simulink model "VSMr_2023b"  (R2023b)
settings: Solver=ode14x  StartTime=0  StopTime=Sim.tend  FixedStep=0.000125  RelTol=4e-4
model workspace (MAT data in the model file):
  nr_vsm = Simulink.Parameter
  nr_vsm.Value = 2
  nr_vsm.DataType = 'int8'
  nr_vsm.Complexity = 'real'
  nr_vsm.Dimensions = [1 1]
values from neighbouring files (symbols this model uses):
  ControlSampleTime = 1/8000    (= 0.000125)    [sim3run_390.m]
  ddfmax = 60    [prm3var_390.m]
  T_seccontrol = 20    [prm3var_390.m]
  Ts = TS    [sim3run_390.m]
  TVRint = 0.85    [prm3var_390.m]
  vsm_Tdaco = 0.01    [prm3var_390.m]
undefined symbols (not defined in the file or in its folder): DiscIntNeverNeededParam, General, parameterset, prm_vsm, pu_vsm, UFLS, VSM
libraries: simulink x55, FriedrichLibrary x10, simulink_extras x2, spsSampleandHoldLib x2
(part 1 of 3)
settings Model: ParameterArgumentNames=nr_vsm  Creator=e2n052  LastModifiedBy=uk062294
settings SolverCC: AlgebraicLoopSolver=TrustRegion
settings DataIOCC: SaveOutput=off  SaveTime=off  ReturnWorkspaceOutputs=off
settings DebuggingCC: UnconnectedInputMsg=warning  UnconnectedOutputMsg=warning  UnconnectedLineMsg=warning  ArithmeticOperatorsInVariantConditions=warning
settings ModelReferenceCC: EnableRefExpFcnMdlSchedulingChecks=on
settings SFSimCC: SimUseLocalCustomCode=off  CustomCodeUndefinedFunction=UseInterfaceOnly
settings RTWCC: RTWUseLocalCustomCode=off  DLArmComputeVersion=19.05
settings GRTTargetCC: CombineOutputUpdateFcns=off  MatFileLogging=off

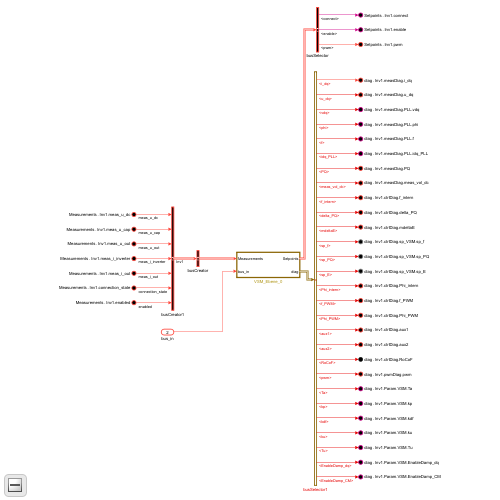
[thumbnail: Simulink's stored preview of the top-level diagram]
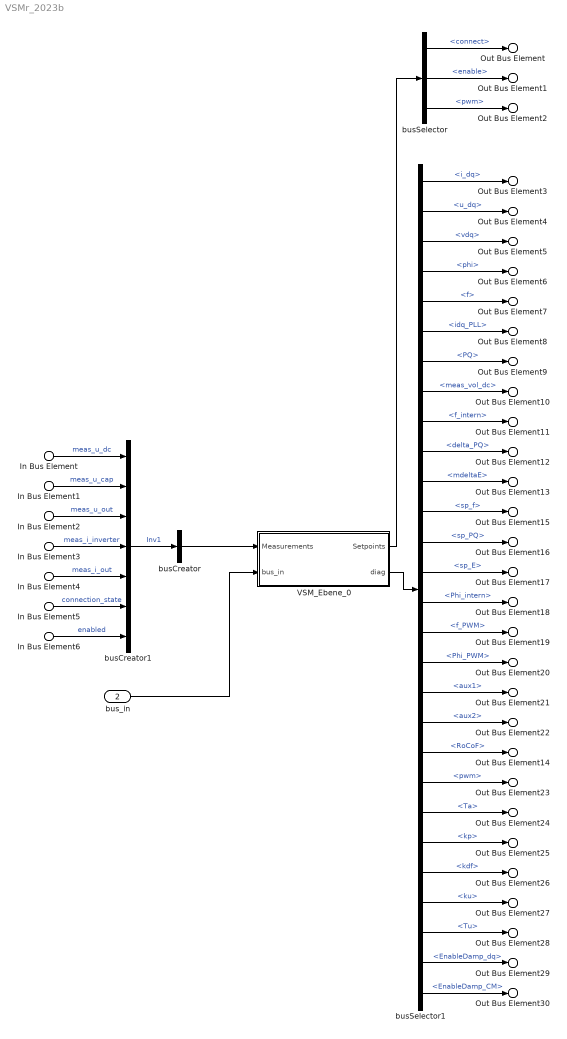
== system VSMr_2023b ==
  In Bus Element : Inport  PortName=Measurements  Element=Inv1.meas_u_dc
  In Bus Element1 : Inport  PortName=Measurements  Element=Inv1.meas_u_cap
  In Bus Element2 : Inport  PortName=Measurements  Element=Inv1.meas_u_out
  In Bus Element3 : Inport  PortName=Measurements  Element=Inv1.meas_i_inverter
  In Bus Element4 : Inport  PortName=Measurements  Element=Inv1.meas_i_out
  In Bus Element5 : Inport  PortName=Measurements  Element=Inv1.connection_state
  In Bus Element6 : Inport  PortName=Measurements  Element=Inv1.enabled
  bus_in : Inport  Port=2
  VSM_Ebene_0 : Subsystem  TreatAsAtomicUnit=on
      settings: MinAlgLoopOccurrences=on
  busCreator : BusCreator  Inputs=1
  busCreator1 : BusCreator  Inputs=7
  busSelector : BusSelector  OutputSignals=Inv1.connect,Inv1.enable,Inv1.pwm
  busSelector1 : BusSelector  OutputSignals=measDiag.i_dq,measDiag.u_dq,measDiag.PLL.vdq,measDiag.PLL.phi,measDiag.PLL.f,measDiag.PLL.idq_PLL,measDiag.PQ,measDiag.meas_vol_dc,ctrlDiag.f_intern,ctrlDiag.delta_PQ,ctrlDiag.mdeltaE,ctrlDiag.sp_VSM.sp_f,ctrlDiag.sp_VSM.sp_PQ,ctrlDiag.sp_VSM.sp_E,ctrlDiag.Phi_intern,ctrlDiag.f_PWM,ctrlDiag.Phi_PWM,ctrlDiag.aux1,ctrlDiag.aux2,ctrlDiag.RoCoF,pwmDiag.pwm,Param.VSM.Ta,Param.VSM.kp,Param.VSM.kdf,Param.VSM.ku,Param.VSM.Tu,Param.VSM.EnableDamp_dq,Param.VSM.EnableDamp_CM
  Out Bus Element : Outport  PortName=Setpoints  Element=Inv1.connect
  Out Bus Element1 : Outport  PortName=Setpoints  Element=Inv1.enable
  Out Bus Element2 : Outport  PortName=Setpoints  Element=Inv1.pwm
  Out Bus Element3 : Outport  Port=2  PortName=diag  Element=Inv1.measDiag.i_dq
  Out Bus Element4 : Outport  Port=2  PortName=diag  Element=Inv1.measDiag.u_dq
  Out Bus Element5 : Outport  Port=2  PortName=diag  Element=Inv1.measDiag.PLL.vdq
  Out Bus Element6 : Outport  Port=2  PortName=diag  Element=Inv1.measDiag.PLL.phi
  Out Bus Element7 : Outport  Port=2  PortName=diag  Element=Inv1.measDiag.PLL.f
  Out Bus Element8 : Outport  Port=2  PortName=diag  Element=Inv1.measDiag.PLL.idq_PLL
  Out Bus Element9 : Outport  Port=2  PortName=diag  Element=Inv1.measDiag.PQ
  Out Bus Element10 : Outport  Port=2  PortName=diag  Element=Inv1.measDiag.meas_vol_dc
  Out Bus Element11 : Outport  Port=2  PortName=diag  Element=Inv1.ctrlDiag.f_intern
  Out Bus Element12 : Outport  Port=2  PortName=diag  Element=Inv1.ctrlDiag.delta_PQ
  Out Bus Element13 : Outport  Port=2  PortName=diag  Element=Inv1.ctrlDiag.mdeltaE
  Out Bus Element15 : Outport  Port=2  PortName=diag  Element=Inv1.ctrlDiag.sp_VSM.sp_f
  Out Bus Element16 : Outport  Port=2  PortName=diag  Element=Inv1.ctrlDiag.sp_VSM.sp_PQ
  Out Bus Element17 : Outport  Port=2  PortName=diag  Element=Inv1.ctrlDiag.sp_VSM.sp_E
  Out Bus Element18 : Outport  Port=2  PortName=diag  Element=Inv1.ctrlDiag.Phi_intern
  Out Bus Element19 : Outport  Port=2  PortName=diag  Element=Inv1.ctrlDiag.f_PWM
  Out Bus Element20 : Outport  Port=2  PortName=diag  Element=Inv1.ctrlDiag.Phi_PWM
  Out Bus Element21 : Outport  Port=2  PortName=diag  Element=Inv1.ctrlDiag.aux1
  Out Bus Element22 : Outport  Port=2  PortName=diag  Element=Inv1.ctrlDiag.aux2
  Out Bus Element14 : Outport  Port=2  PortName=diag  Element=Inv1.ctrlDiag.RoCoF
  Out Bus Element23 : Outport  Port=2  PortName=diag  Element=Inv1.pwmDiag.pwm
  Out Bus Element24 : Outport  Port=2  PortName=diag  Element=Inv1.Param.VSM.Ta
  Out Bus Element25 : Outport  Port=2  PortName=diag  Element=Inv1.Param.VSM.kp
  Out Bus Element26 : Outport  Port=2  PortName=diag  Element=Inv1.Param.VSM.kdf
  Out Bus Element27 : Outport  Port=2  PortName=diag  Element=Inv1.Param.VSM.ku
  Out Bus Element28 : Outport  Port=2  PortName=diag  Element=Inv1.Param.VSM.Tu
  Out Bus Element29 : Outport  Port=2  PortName=diag  Element=Inv1.Param.VSM.EnableDamp_dq
  Out Bus Element30 : Outport  Port=2  PortName=diag  Element=Inv1.Param.VSM.EnableDamp_CM
  wires:
  busSelector1/27 -> Out Bus Element29/1  "<EnableDamp_dq>"
  busSelector1/25 -> Out Bus Element27/1  "<ku>"
  busSelector1/23 -> Out Bus Element25/1  "<kp>"
  busSelector1/21 -> Out Bus Element23/1  "<pwm>"
  busSelector1/28 -> Out Bus Element30/1  "<EnableDamp_CM>"
  busSelector1/26 -> Out Bus Element28/1  "<Tu>"
  busSelector1/24 -> Out Bus Element26/1  "<kdf>"
  busSelector1/22 -> Out Bus Element24/1  "<Ta>"
  busSelector1/13 -> Out Bus Element16/1  "<sp_PQ>"
  busSelector1/15 -> Out Bus Element18/1  "<Phi_intern>"
  busSelector1/17 -> Out Bus Element20/1  "<Phi_PWM>"
  busSelector1/19 -> Out Bus Element22/1  "<aux2>"
  busSelector1/12 -> Out Bus Element15/1  "<sp_f>"
  busSelector1/14 -> Out Bus Element17/1  "<sp_E>"
  busSelector1/16 -> Out Bus Element19/1  "<f_PWM>"
  busSelector1/18 -> Out Bus Element21/1  "<aux1>"
  busSelector1/6 -> Out Bus Element8/1  "<idq_PLL>"
  busSelector1/8 -> Out Bus Element10/1  "<meas_vol_dc>"
  busSelector1/10 -> Out Bus Element12/1  "<delta_PQ>"
  busSelector1/5 -> Out Bus Element7/1  "<f>"
  busSelector1/7 -> Out Bus Element9/1  "<PQ>"
  busSelector1/9 -> Out Bus Element11/1  "<f_intern>"
  busSelector1/11 -> Out Bus Element13/1  "<mdeltaE>"
  busSelector1/2 -> Out Bus Element4/1  "<u_dq>"
  busSelector1/4 -> Out Bus Element6/1  "<phi>"
  busSelector1/1 -> Out Bus Element3/1  "<i_dq>"
  busSelector1/3 -> Out Bus Element5/1  "<vdq>"
  busCreator/1 -> VSM_Ebene_0/1(Measurements)
  VSM_Ebene_0/2(diag) -> busSelector1/1
  In Bus Element6/1 -> busCreator1/7  "enabled"
  busSelector/1 -> Out Bus Element/1  "<connect>"
  busSelector/3 -> Out Bus Element2/1  "<pwm>"
  busSelector/2 -> Out Bus Element1/1  "<enable>"
  In Bus Element3/1 -> busCreator1/4  "meas_i_inverter"
  In Bus Element5/1 -> busCreator1/6  "connection_state"
  In Bus Element4/1 -> busCreator1/5  "meas_i_out"
  In Bus Element2/1 -> busCreator1/3  "meas_u_out"
  In Bus Element1/1 -> busCreator1/2  "meas_u_cap"
  In Bus Element/1 -> busCreator1/1  "meas_u_dc"
  busCreator1/1 -> busCreator/1  "Inv1"
  bus_in/1 -> VSM_Ebene_0/2(bus_in)
  VSM_Ebene_0/1(Setpoints) -> busSelector/1
  busSelector1/20 -> Out Bus Element14/1  "<RoCoF>"

== system VSMr_2023b/VSM_Ebene_0 ==
  Measurements : Inport
  bus_in : Inport  Port=2
  Constant : Constant  Value=prm_vsm{51,nr_vsm}
  VSM_Ebene_1 : Subsystem  DialogController=POWERSYS.PowerSysDialog
  command_center0 : Subsystem
  sp_E0 : Constant  Value=prm_vsm{32,nr_vsm}
  sp_P1 : Constant  Value=prm_vsm{1, nr_vsm}  VectorParams1D=off
  Setpoints : Outport
  diag : Outport  Port=2
  wires:
  Measurements/1 -> VSM_Ebene_1/1(Measurements)
  Constant/1 -> command_center0/2(Qref)
  sp_P1/1 -> command_center0/1(Pref)
  VSM_Ebene_1/2(diag) -> diag/1
  VSM_Ebene_1/1(Setpoints) -> Setpoints/1
  command_center0/1(cmd_ac) -> VSM_Ebene_1/2("cmd ")
  sp_E0/1 -> command_center0/3(Eref)
  bus_in/1 -> VSM_Ebene_1/3(bus_in)

== system VSMr_2023b/VSM_Ebene_0/VSM_Ebene_1 ==
  Measurements : Inport
  "cmd " : Inport  Port=2
  bus_in : Inport  Port=3
  Bus Creator : BusCreator  Inputs=1
  Bus Selector2 : BusSelector  OutputSignals=Inv1
  VSM_Ebene_2 : Subsystem
  Setpoints : Outport  VectorParamsAs1DForOutWhenUnconnected=off
  diag : Outport  Port=2  VectorParamsAs1DForOutWhenUnconnected=off
  wires:
  Measurements/1 -> Bus Selector2/1
  Bus Selector2/1 -> VSM_Ebene_2/2(meas)  "<Inv1>"
  VSM_Ebene_2/2(diag) -> [inv1diag]
  [inv1diag] -> diag/1  "Inv1"
  Bus Creator/1 -> Setpoints/1
  VSM_Ebene_2/1(ctrl) -> Bus Creator/1  "Inv1"
  "cmd "/1 -> VSM_Ebene_2/1(cmd)
  bus_in/1 -> VSM_Ebene_2/3(f_ufls)

== system VSMr_2023b/VSM_Ebene_0/command_center0 ==
  Pref : Inport
  Qref : Inport  Port=2
  Eref : Inport  Port=3
  Bus Creator1 : BusCreator  Inputs=1
  Bus Creator3 : BusCreator  Inputs=7
  Bus Creator4 : BusCreator  Inputs=3
  Bus Creator15 : BusCreator  Inputs=5
  Constant : Constant
  Constant4 : Constant
  Constant5 : Constant
  EnableDamp_CM [0/1] : Constant  Value=0
  EnableDamp_dq [0/1] : Constant
  Mux : Mux  Inputs=2
  Ta : Constant  Value=0
  Ta1 : Constant  Value=0
  Ta2 : Constant  Value=prm_vsm{25, nr_vsm}
  Ta3 : Constant  Value=prm_vsm{26, nr_vsm}
  Ta4 : Constant  Value=prm_vsm{27, nr_vsm}
  sp_f [Hz] : Constant  Value=50
  cmd_ac : Outport  VectorParamsAs1DForOutWhenUnconnected=off
  wires:
  Bus Creator15/1 -> cmd_ac/1
  Constant4/1 -> Bus Creator15/2  "connect"
  Constant/1 -> Bus Creator15/1  "preload"
  Bus Creator1/1 -> Bus Creator15/5  "Param"
  Constant5/1 -> Bus Creator15/3  "enable"
  Ta/1 -> Bus Creator3/1  "Ta"
  Bus Creator3/1 -> Bus Creator1/1  "VSM"
  Ta2/1 -> Bus Creator3/3  "kdf"
  Ta1/1 -> Bus Creator3/2  "kp"
  Ta3/1 -> Bus Creator3/4  "ku"
  Ta4/1 -> Bus Creator3/5  "Tu"
  Bus Creator4/1 -> Bus Creator15/4  "sp_VSM"
  sp_f [Hz]/1 -> Bus Creator4/1  "sp_f"
  Mux/1 -> Bus Creator4/2  "sp_PQ"
  Eref/1 -> Bus Creator4/3  "sp_E"
  EnableDamp_dq [0/1]/1 -> Bus Creator3/6  "EnableDamp_dq"
  EnableDamp_CM [0/1]/1 -> Bus Creator3/7  "EnableDamp_CM"
  Qref/1 -> Mux/2
  Pref/1 -> Mux/1

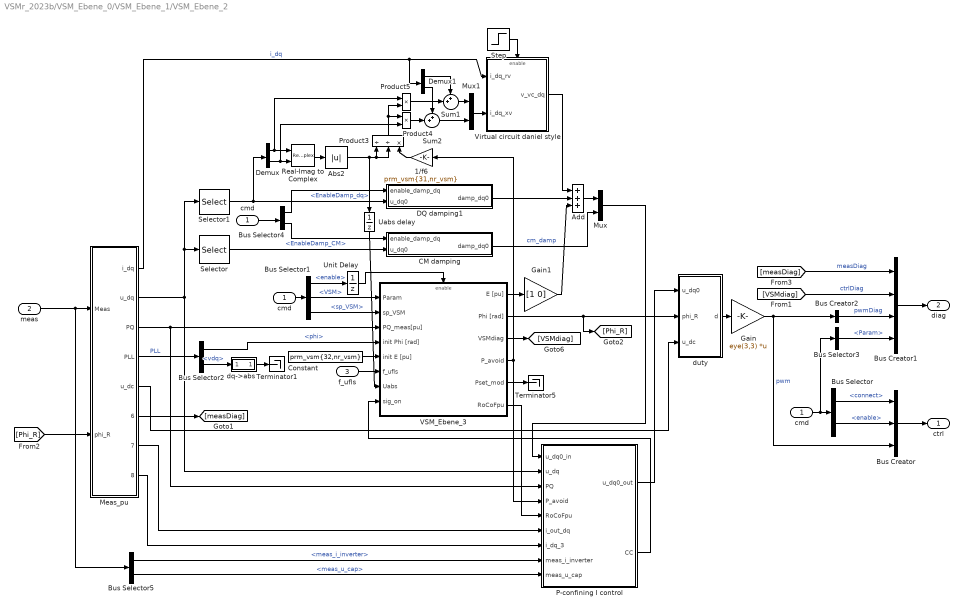
== system VSMr_2023b/VSM_Ebene_0/VSM_Ebene_1/VSM_Ebene_2 ==
  cmd : Inport
  meas : Inport  Port=2
  f_ufls : Inport  Port=3
  " cmd " : InportShadow
  1/f6 : Gain  Gain=prm_vsm{31,nr_vsm}
  Abs2 : Abs  SaturateOnIntegerOverflow=off
  Add : Sum  Inputs=+++
  Bus Creator : BusCreator  Inputs=3
  Bus Creator1 : BusCreator  Inputs=4
  Bus Creator2 : BusCreator  Inputs=1
  Bus Selector : BusSelector  OutputSignals=connect,enable
  Bus Selector1 : BusSelector  OutputSignals=enable,Param.VSM,sp_VSM
  Bus Selector2 : BusSelector  OutputSignals=phi,vdq
  Bus Selector3 : BusSelector  OutputSignals=Param
  Bus Selector4 : BusSelector  OutputSignals=Param.VSM.EnableDamp_dq,Param.VSM.EnableDamp_CM
  Bus Selector5 : BusSelector  OutputSignals=meas_i_inverter,meas_u_cap
  CM damping : Subsystem  mask(Lead Lag){OmLead=prm_vsm{11,nr_vsm}, OmLag=prm_vsm{12,nr_vsm}}
      mask prompts: OmLead "Omega Lead"; OmLag "Omega Lag"
  Constant : Constant  Value=prm_vsm{32,nr_vsm}
  DQ damping1 : Subsystem  mask(Lead Lag){OmLead=prm_vsm{11,nr_vsm}, OmLag=prm_vsm{12,nr_vsm}}
      mask prompts: OmLead "Omega Lead"; OmLag "Omega Lag"
  Demux : Demux  Outputs=2
  Demux1 : Demux  Outputs=2
  Gain : Gain  Gain=eye(3,3)  Multiplication=Matrix(K*u)
  Gain1 : Gain  Gain=[1 0]
  Meas_pu : Subsystem
  Mux : Mux  Inputs=[2 1]
  Mux1 : Mux  Inputs=2
  P-confining I control : Subsystem
  Product3 : Product  Inputs=//*
  Product4 : Product
  Product5 : Product
  Real-Imag to Complex : RealImagToComplex
  Selector : Selector  InputPortWidth=3  IndexOptions=Index vector (dialog)  Indices=[3]  OutputSizes=1
  Selector1 : Selector  InputPortWidth=3  IndexOptions=Index vector (dialog)  Indices=[1 2]  OutputSizes=1
  Step : Step  Time=0.001  SampleTime=0
  Sum1 : Sum  Inputs=++|
  Sum2 : Sum  Inputs=++|
  Terminator1 : Terminator
  Terminator5 : Terminator
  Uabs delay : UnitDelay  InitialCondition=1  SampleTime=-1  HasFrameUpgradeWarning=on
  Unit Delay : UnitDelay  SampleTime=ControlSampleTime  HasFrameUpgradeWarning=on
  VSM_Ebene_3 : Subsystem
  Virtual circuit daniel style : Subsystem
  "cmd " : InportShadow
  dq->abs : Subsystem
  duty : Subsystem
  ctrl : Outport  VectorParamsAs1DForOutWhenUnconnected=off
  diag : Outport  Port=2  VectorParamsAs1DForOutWhenUnconnected=off
  wires:
  Unit Delay/1 -> VSM_Ebene_3/Enable
  Product3/1 -> Product4/1, Product5/2
  Bus Selector1/3 -> VSM_Ebene_3/2(sp_VSM)  "<sp_VSM>"
  Demux/2 -> Real-Imag to Complex/2, Product4/2
  Demux/1 -> Real-Imag to Complex/1, Product5/1
  Selector1/1 -> Demux/1, DQ damping1/2(u_dq0)
  Real-Imag to Complex/1 -> Abs2/1
  Step/1 -> Virtual circuit daniel style/Enable
  Mux1/1 -> Virtual circuit daniel style/2(i_dq_xv)
  Demux1/1 -> Sum1/1
  Sum2/1 -> Mux1/2
  Demux1/2 -> Sum2/1
  Sum1/1 -> Mux1/1
  Product5/1 -> Sum1/2
  Bus Creator2/1 -> Bus Creator1/3  "pwmDiag"
  Bus Selector3/1 -> Bus Creator1/4  "<Param>"
  cmd/1 -> Bus Selector3/1, Bus Selector/1
  Bus Selector1/1 -> Unit Delay/1  "<enable>"
  Bus Creator1/1 -> diag/1
  [VSMdiag] -> Bus Creator1/2  "ctrlDiag"
  [measDiag] -> Bus Creator1/1  "measDiag"
  Gain/1 -> Bus Creator2/1, Bus Creator/3  "pwm"
  Bus Selector/2 -> Bus Creator/2  "<enable>"
  Bus Creator/1 -> ctrl/1
  Bus Selector/1 -> Bus Creator/1  "<connect>"
  Meas_pu/6(measDiag) -> [measDiag]
  Bus Selector1/2 -> VSM_Ebene_3/1(Param)  "<VSM>"
  VSM_Ebene_3/2(Phi [rad]) -> duty/2(phi_R), [Phi_R]
  [Phi_R] -> Meas_pu/2(phi_R)
  Meas_pu/4(PLL) -> Bus Selector2/1  "PLL"
  Bus Selector2/2 -> dq->abs/1(In1)  "<vdq>"
  VSM_Ebene_3/3(VSMdiag) -> [VSMdiag]
  Bus Selector2/1 -> VSM_Ebene_3/4(init Phi [rad])  "<phi>"
  Selector/1 -> CM damping/2(u_dq0)
  CM damping/1(damp_dq0) -> Mux/2  "cm_damp"
  Add/1 -> Mux/1
  Bus Selector4/1 -> DQ damping1/1(enable_damp_dq)  "<EnableDamp_dq>"
  Bus Selector4/2 -> CM damping/1(enable_damp_dq)  "<EnableDamp_CM>"
  " cmd "/1 -> Bus Selector4/1
  "cmd "/1 -> Bus Selector1/1
  Meas_pu/5(u_dc) -> duty/3(u_dc)
  dq->abs/1(abs) -> Terminator1/1
  Constant/1 -> VSM_Ebene_3/5(init E [pu])
  VSM_Ebene_3/1(E [pu]) -> Gain1/1
  Uabs delay/1 -> VSM_Ebene_3/7(Uabs)
  f_ufls/1 -> VSM_Ebene_3/6(f_ufls)
  duty/1(d) -> Gain/1
  Product4/1 -> Sum2/2
  Meas_pu/3(PQ) -> VSM_Ebene_3/3(PQ_meas[pu]), P-confining I control/3(PQ)
  meas/1 -> Bus Selector5/1, Meas_pu/1(Meas)
  Meas_pu/2(u_dq) -> P-confining I control/2(u_dq), Selector1/1, Selector/1
  Meas_pu/1(i_dq) -> Demux1/1, Virtual circuit daniel style/1(i_dq_rv)  "i_dq"
  Abs2/1 -> Product3/2, Product3/1, Uabs delay/1
  Virtual circuit daniel style/1(v_vc_dq) -> Add/1
  Gain1/1 -> Add/3
  DQ damping1/1(damp_dq0) -> Add/2
  1/f6/1 -> Product3/3
  VSM_Ebene_3/5(Pset_mod) -> Terminator5/1
  VSM_Ebene_3/4(P_avoid) -> P-confining I control/4(P_avoid), 1/f6/1
  Mux/1 -> P-confining I control/1(u_dq0_in)
  VSM_Ebene_3/6(RoCoFpu) -> P-confining I control/5(RoCoFpu)
  Meas_pu/7(i_out_dq) -> P-confining I control/6(i_out_dq)
  Meas_pu/8(i_dq_3) -> P-confining I control/7(i_dq_3)
  Bus Selector5/1 -> P-confining I control/8(meas_i_inverter)  "<meas_i_inverter>"
  Bus Selector5/2 -> P-confining I control/9(meas_u_cap)  "<meas_u_cap>"
  P-confining I control/1(u_dq0_out) -> duty/1(u_dq0)
  P-confining I control/2(CC) -> VSM_Ebene_3/8(sig_on)

== system VSMr_2023b/VSM_Ebene_0/VSM_Ebene_1/VSM_Ebene_2/CM damping ==
  enable_damp_dq : Inport
  u_dq0 : Inport  Port=2
  Gain2 : Gain  Gain=OmLead
  Gain5 : Gain  Gain=OmLag
  Integrator (inertia) : DiscreteIntegrator  gainval=1  InitialCondition=1  SampleTime=ControlSampleTime  ICPrevOutput=DiscIntNeverNeededParam  ICPrevScaledInput=DiscIntNeverNeededParam
  Product : Product
  Product1 : Product
  Sum : Sum  Inputs=|+-
  Sum2 : Sum  Inputs=++|
  damp_dq0 : Outport  VectorParamsAs1DForOutWhenUnconnected=off
  wires:
  Gain2/1 -> Sum/1
  Integrator (inertia)/1 -> Sum2/2
  Gain5/1 -> Sum/2
  Sum2/1 -> Product1/2, Gain5/1
  Sum/1 -> Integrator (inertia)/1
  u_dq0/1 -> Product/2
  Product/1 -> Sum2/1, Gain2/1
  enable_damp_dq/1 -> Product1/1, Product/1
  Product1/1 -> damp_dq0/1

== system VSMr_2023b/VSM_Ebene_0/VSM_Ebene_1/VSM_Ebene_2/DQ damping1 ==
  enable_damp_dq : Inport
  u_dq0 : Inport  Port=2
  Gain2 : Gain  Gain=OmLead
  Gain5 : Gain  Gain=OmLag
  Integrator (inertia) : DiscreteIntegrator  gainval=1  InitialCondition=1  SampleTime=ControlSampleTime  ICPrevOutput=DiscIntNeverNeededParam  ICPrevScaledInput=DiscIntNeverNeededParam
  Product : Product
  Product1 : Product
  Sum : Sum  Inputs=|+-
  Sum2 : Sum  Inputs=++|
  damp_dq0 : Outport  VectorParamsAs1DForOutWhenUnconnected=off
  wires:
  Product1/1 -> damp_dq0/1
  enable_damp_dq/1 -> Product/1, Product1/1
  Product/1 -> Gain2/1, Sum2/1
  u_dq0/1 -> Product/2
  Sum/1 -> Integrator (inertia)/1
  Sum2/1 -> Gain5/1, Product1/2
  Gain5/1 -> Sum/2
  Integrator (inertia)/1 -> Sum2/2
  Gain2/1 -> Sum/1

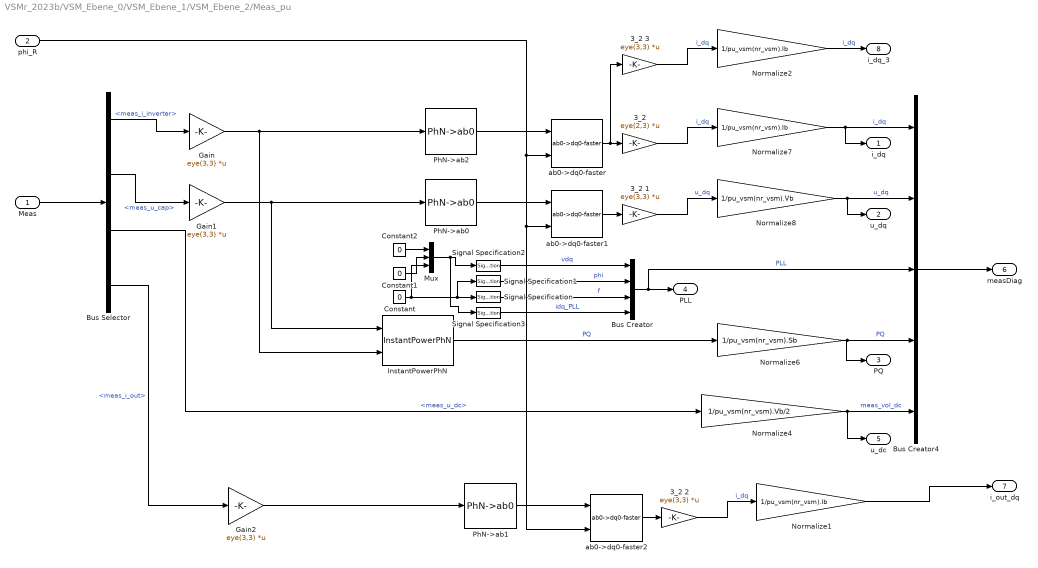
== system VSMr_2023b/VSM_Ebene_0/VSM_Ebene_1/VSM_Ebene_2/Meas_pu ==
  Meas : Inport
  phi_R : Inport  Port=2
  "3_2 " : Gain  Gain=eye(2,3)  Multiplication=Matrix(K*u)
  3_2 1 : Gain  Gain=eye(3,3)  Multiplication=Matrix(K*u)
  3_2 2 : Gain  Gain=eye(3,3)  Multiplication=Matrix(K*u)
  3_2 3 : Gain  Gain=eye(3,3)  Multiplication=Matrix(K*u)
  Bus Creator : BusCreator  Inputs=4
  Bus Creator4 : BusCreator  Inputs=5
  Bus Selector : BusSelector  OutputSignals=meas_i_inverter,meas_u_cap,meas_u_dc,meas_i_out
  Constant : Constant  Value=0
  Constant1 : Constant  Value=0
  Constant2 : Constant  Value=0
  Gain : Gain  Gain=eye(3,3)  Multiplication=Matrix(K*u)
  Gain1 : Gain  Gain=eye(3,3)  Multiplication=Matrix(K*u)
  Gain2 : Gain  Gain=eye(3,3)  Multiplication=Matrix(K*u)
  InstantPowerPhN : FriedrichLibrary/Transformations/InstantPowerPhN  SystemSampleTime=-1  VariantActivationTime=update diagram  AllowFlexibleInterface=on  Latency=0  AutoFrameSizeCalculation=off
  Mux : Mux  Inputs=3
  Normalize1 : Gain  Gain=1/pu_vsm(nr_vsm).Ib  OutDataTypeStr=double  RndMeth=Round
  Normalize2 : Gain  Gain=1/pu_vsm(nr_vsm).Ib  OutDataTypeStr=double  RndMeth=Round
  Normalize4 : Gain  Gain=1/pu_vsm(nr_vsm).Vb/2  OutDataTypeStr=double  RndMeth=Round
  Normalize6 : Gain  Gain=1/pu_vsm(nr_vsm).Sb  OutDataTypeStr=double  RndMeth=Round
  Normalize7 : Gain  Gain=1/pu_vsm(nr_vsm).Ib  OutDataTypeStr=double  RndMeth=Round
  Normalize8 : Gain  Gain=1/pu_vsm(nr_vsm).Vb  OutDataTypeStr=double  RndMeth=Round
  PhN->ab0 : FriedrichLibrary/Transformations/PhN->ab0  SystemSampleTime=-1  VariantActivationTime=update diagram  AllowFlexibleInterface=on  Latency=0  AutoFrameSizeCalculation=off
  PhN->ab1 : FriedrichLibrary/Transformations/PhN->ab0  SystemSampleTime=-1  VariantActivationTime=update diagram  AllowFlexibleInterface=on  Latency=0  AutoFrameSizeCalculation=off
  PhN->ab2 : FriedrichLibrary/Transformations/PhN->ab0  SystemSampleTime=-1  VariantActivationTime=update diagram  AllowFlexibleInterface=on  Latency=0  AutoFrameSizeCalculation=off
  Signal Specification : SignalSpecification  Dimensions=1
  Signal Specification1 : SignalSpecification  Dimensions=1
  Signal Specification2 : SignalSpecification  Dimensions=3
  Signal Specification3 : SignalSpecification  Dimensions=3
  ab0->dq0-faster : FriedrichLibrary/Transformations/ab0->dq0-faster  SystemSampleTime=-1  VariantActivationTime=update diagram  AllowFlexibleInterface=on  Latency=0  AutoFrameSizeCalculation=off
  ab0->dq0-faster1 : FriedrichLibrary/Transformations/ab0->dq0-faster  SystemSampleTime=-1  VariantActivationTime=update diagram  AllowFlexibleInterface=on  Latency=0  AutoFrameSizeCalculation=off
  ab0->dq0-faster2 : FriedrichLibrary/Transformations/ab0->dq0-faster  SystemSampleTime=-1  VariantActivationTime=update diagram  AllowFlexibleInterface=on  Latency=0  AutoFrameSizeCalculation=off
  i_dq : Outport  VectorParamsAs1DForOutWhenUnconnected=off
  u_dq : Outport  Port=2  VectorParamsAs1DForOutWhenUnconnected=off
  PQ : Outport  Port=3  VectorParamsAs1DForOutWhenUnconnected=off
  PLL : Outport  Port=4  VectorParamsAs1DForOutWhenUnconnected=off
  u_dc : Outport  Port=5  VectorParamsAs1DForOutWhenUnconnected=off
  measDiag : Outport  Port=6  VectorParamsAs1DForOutWhenUnconnected=off
  i_out_dq : Outport  Port=7  VectorParamsAs1DForOutWhenUnconnected=off
  i_dq_3 : Outport  Port=8  VectorParamsAs1DForOutWhenUnconnected=off
  wires:
  Mux/1 -> Signal Specification2/1, Signal Specification3/1
  Constant1/1 -> Mux/2
  Constant2/1 -> Mux/1
  Constant/1 -> Mux/3, Signal Specification/1, Signal Specification1/1
  Normalize8/1 -> Bus Creator4/2, u_dq/1  "u_dq"
  Normalize7/1 -> Bus Creator4/1, i_dq/1  "i_dq"
  Normalize6/1 -> PQ/1, Bus Creator4/4  "PQ"
  InstantPowerPhN/1 -> Normalize6/1  "PQ"
  Gain1/1 -> InstantPowerPhN/1, PhN->ab0/1
  Gain/1 -> InstantPowerPhN/2, PhN->ab2/1
  "3_2 "/1 -> Normalize7/1  "i_dq"
  3_2 1/1 -> Normalize8/1  "u_dq"
  Bus Creator/1 -> Bus Creator4/3, PLL/1  "PLL"
  Bus Selector/2 -> Gain1/1  "<meas_u_cap>"
  ab0->dq0-faster1/1 -> 3_2 1/1
  PhN->ab2/1 -> ab0->dq0-faster/1
  PhN->ab0/1 -> ab0->dq0-faster1/1
  Bus Selector/1 -> Gain/1  "<meas_i_inverter>"
  Bus Selector/3 -> Normalize4/1  "<meas_u_dc>"
  Meas/1 -> Bus Selector/1
  Bus Creator4/1 -> measDiag/1
  Signal Specification/1 -> Bus Creator/3  "f"
  Signal Specification1/1 -> Bus Creator/2  "phi"
  Signal Specification2/1 -> Bus Creator/1  "vdq"
  Signal Specification3/1 -> Bus Creator/4  "idq_PLL"
  Normalize4/1 -> u_dc/1, Bus Creator4/5  "meas_vol_dc"
  phi_R/1 -> ab0->dq0-faster2/2, ab0->dq0-faster1/2, ab0->dq0-faster/2
  Normalize1/1 -> i_out_dq/1
  Gain2/1 -> PhN->ab1/1
  PhN->ab1/1 -> ab0->dq0-faster2/1
  ab0->dq0-faster2/1 -> 3_2 2/1
  3_2 2/1 -> Normalize1/1  "i_dq"
  Bus Selector/4 -> Gain2/1  "<meas_i_out>"
  3_2 3/1 -> Normalize2/1  "i_dq"
  Normalize2/1 -> i_dq_3/1  "i_dq"
  ab0->dq0-faster/1 -> 3_2 3/1, "3_2 "/1

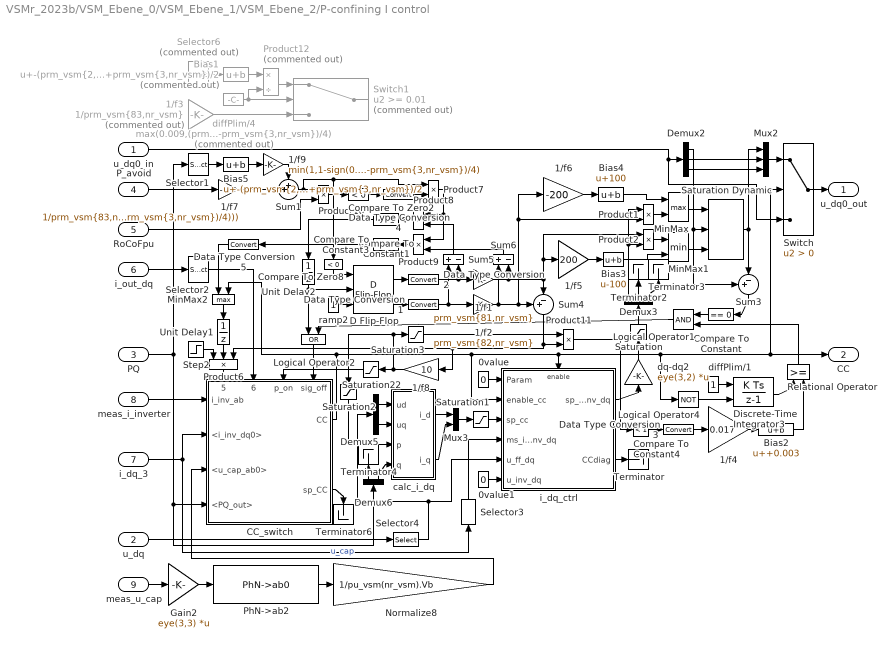
== system VSMr_2023b/VSM_Ebene_0/VSM_Ebene_1/VSM_Ebene_2/P-confining I control ==
  u_dq0_in : Inport
  u_dq : Inport  Port=2
  PQ : Inport  Port=3
  P_avoid : Inport  Port=4
  RoCoFpu : Inport  Port=5
  i_out_dq : Inport  Port=6
  i_dq_3 : Inport  Port=7
  meas_i_inverter : Inport  Port=8
  meas_u_cap : Inport  Port=9
  0value : Constant  Value=0
  0value1 : Constant  Value=0
  1/f1 : Gain  Gain=prm_vsm{81,nr_vsm}
  1/f2 : Gain  Gain=prm_vsm{82,nr_vsm}
  1/f3 : Gain  Commented=on  Gain=1/prm_vsm{83,nr_vsm}
  1/f4 : Gain  Gain=0.017
  1/f5 : Gain  Gain=200
  1/f6 : Gain  Gain=-200
  1/f7 : Gain  Gain=1/prm_vsm{83,nr_vsm}*max(0,sign(0.01-max(0.009,(prm_vsm{2,nr_vsm}-prm_vsm{3,nr_vsm})/4)))
  1/f8 : Gain  Gain=10
  1/f9 : Gain  Gain=min(1,1-sign(0.01-max(0.009,(prm_vsm{2,nr_vsm}-prm_vsm{3,nr_vsm})/4)))/max(0.009,(prm_vsm{2,nr_vsm}-prm_vsm{3,nr_vsm})/4)
  Bias1 : Bias  Commented=on  Bias=-(prm_vsm{2,nr_vsm}+prm_vsm{3,nr_vsm})/2  SaturateOnIntegerOverflow=off
  Bias2 : Bias  Bias=+0.003  SaturateOnIntegerOverflow=off
  Bias3 : Bias  Bias=-100  SaturateOnIntegerOverflow=off
  Bias4 : Bias  Bias=100  SaturateOnIntegerOverflow=off
  Bias5 : Bias  Bias=-(prm_vsm{2,nr_vsm}+prm_vsm{3,nr_vsm})/2  SaturateOnIntegerOverflow=off
  CC_switch : Subsystem
      settings: PortSchema="{\"entries\":[{\"content\":{\"sides\":[{\"content\":{\"connectorIds\":[\"In1\",\"In2\",\"In3\",\"In4\"]},\"type\":\"ConnectorPlacement.EquallySpacedRectSide\",\"uuid\":\"aab35d75-627c-4ffd-9951-e3576d7320db\"},{\"content\":{\"connectorIds\":[\"Out1\",\"Out2\"],\"side\":\"RIGHT\"},\"type\":\"ConnectorPlacement.EquallySpacedRectSide\",\"uuid\":\"99390366-615d-4dc0-a4b9-7a01bc996075\"},{\"content\":{\"connectorIds\":[\"In5\",\"In6\",\"In7\",\"In8\"],\"side\":\"TOP\"},\"type\":\"ConnectorPlacement.EquallySpacedRectSide\",\"uuid\":\"cd480ac8-3fd2-414e-8b74-691c5964b8fa\"},{\"content\":{\"side\":\"HIDDEN\"},\"type\":\"ConnectorPlacement.EquallySpacedRectSide\",\"uuid\":\"eb094f38-97b3-4aba-ac5e-ab488d071caa\"}]},\"type\":\"ConnectorPlacement.EquallySpacedConnector\",\"uuid\":\"65637395-8c41-4247-973f-480dfd8a7bba\"}],\"packageUris\":[\"http://schema.mathworks.com/mf0/Connector/R2020b\"],\"version\":\"1.0\"}"
  Compare To Constant : simulink/Logic and Bit Operations/Compare To Constant  relop===  const=0  OutDataTypeStr=boolean
  Compare To Constant1 : simulink/Logic and Bit Operations/Compare To Constant  relop=<  const=-1  OutDataTypeStr=boolean
  Compare To Constant3 : simulink/Logic and Bit Operations/Compare To Constant  relop=>  const=1  OutDataTypeStr=boolean
  Compare To Constant4 : simulink/Logic and Bit Operations/Compare To Constant  relop=<  const=1  OutDataTypeStr=boolean
  Compare To Zero2 : simulink/Logic and Bit Operations/Compare To Zero  relop=<  OutDataTypeStr=boolean
  Compare To Zero8 : simulink/Logic and Bit Operations/Compare To Zero  relop=<  OutDataTypeStr=boolean
  D Flip-Flop : simulink_extras/Flip Flops/D Flip-Flop
  Data Type Conversion{1..5} (5 alike) : DataTypeConversion  SaturateOnIntegerOverflow=off  RndMeth=Floor
  Demux2 : Demux  Outputs=3
  Demux3 : Demux  Outputs=3
  Demux5 : Demux  Outputs=2
  Demux6 : Demux  Outputs=2
  Discrete-Time Integrator3 : DiscreteIntegrator  gainval=1  ExternalReset=level  SampleTime=-1  UpperSaturationLimit=0.008  LowerSaturationLimit=0  ICPrevOutput=DiscIntNeverNeededParam  ICPrevScaledInput=DiscIntNeverNeededParam
  Gain2 : Gain  Gain=eye(3,3)  Multiplication=Matrix(K*u)
  Logical Operator1 : Logic  AllPortsSameDT=off  OutDataTypeStr=boolean
  Logical Operator2 : Logic  Operator=OR  AllPortsSameDT=off  OutDataTypeStr=boolean
  Logical Operator4 : Logic  Operator=NOT  AllPortsSameDT=off  OutDataTypeStr=boolean
  MinMax : MinMax  Function=max  Inputs=2
  MinMax1 : MinMax  Inputs=2
  MinMax2 : MinMax  Function=max  Inputs=2
  Mux2 : Mux  Inputs=3
  Mux3 : Mux  Inputs=[1 1]
  Normalize8 : Gain  Gain=1/pu_vsm(nr_vsm).Vb  OutDataTypeStr=double  RndMeth=Round
  PhN->ab2 : FriedrichLibrary/Transformations/PhN->ab0  SystemSampleTime=-1  VariantActivationTime=update diagram  AllowFlexibleInterface=on  Latency=0  AutoFrameSizeCalculation=off
  Product{1..2,7..11} (7 alike) : Product
  Product12 : Product  Commented=on  Inputs=*/
  Product6 : Product  Inputs=3
  Relational Operator : RelationalOperator  OutDataTypeStr=boolean  RndMeth=Simplest  InputSameDT=off
  Saturation : Saturate  UpperLimit=2  LowerLimit=-2
  Saturation Dynamic : simulink/Discontinuities/Saturation Dynamic  OutMin=[]  OutMax=[]  OutDataTypeStr=Inherit: Same as second input  OutDataType=fixdt(1, 16)  OutScaling=2^-10  DoSatur=off
  Saturation1 : Saturate  UpperLimit=2  LowerLimit=-2
  Saturation2 : Saturate  UpperLimit=prm_vsm{2,nr_vsm}+0.005  LowerLimit=prm_vsm{3,nr_vsm}-0.005
  Saturation22 : Saturate  UpperLimit=prm_vsm{2,nr_vsm}+prm_vsm{83,nr_vsm}  LowerLimit=prm_vsm{3,nr_vsm}-prm_vsm{83,nr_vsm}
  Saturation3 : Saturate  UpperLimit=prm_vsm{5,nr_vsm}+0.9  LowerLimit=prm_vsm{4,nr_vsm}-0.9
  Selector1 : Selector  InputPortWidth=2  IndexOptions=Index vector (dialog)  Indices=1  OutputSizes=1
  Selector2 : Selector  InputPortWidth=3  IndexOptions=Index vector (dialog)  Indices=[1 2]  OutputSizes=1
  Selector3 : Selector  InputPortWidth=3  IndexOptions=Index vector (dialog)  Indices=[1 2]  OutputSizes=1
  Selector4 : Selector  InputPortWidth=3  IndexOptions=Index vector (dialog)  Indices=[1 2]  OutputSizes=1
  Selector6 : Selector  Commented=on  InputPortWidth=2  IndexOptions=Index vector (dialog)  Indices=1  OutputSizes=1
  Step2 : Step  Time=1.9  SampleTime=0
  Sum1 : Sum  Inputs=++|
  Sum3 : Sum  Inputs=+-|
  Sum4 : Sum  Inputs=+-|
  Sum5 : Sum  Inputs=+-
  Sum6 : Sum  Inputs=+-
  Switch : Switch  Criteria=u2 > Threshold  SaturateOnIntegerOverflow=off  InputSameDT=off
  Switch1 : Switch  Commented=on  Threshold=0.01  SaturateOnIntegerOverflow=off  InputSameDT=off
  Terminator{,2..4,6} (5 alike) : Terminator
  Unit Delay1 : UnitDelay  SampleTime=ControlSampleTime  HasFrameUpgradeWarning=on
  Unit Delay2 : UnitDelay  SampleTime=ControlSampleTime  HasFrameUpgradeWarning=on
  calc_i_dq : MATLAB Function  TreatAsAtomicUnit=on
  diffPlim/1 : Constant
  diffPlim/4 : Constant  Commented=on  Value=max(0.009,(prm_vsm{2,nr_vsm}-prm_vsm{3,nr_vsm})/4)
  dq-dq2 : Gain  Gain=eye(3,2)  Multiplication=Matrix(K*u)
  i_dq_ctrl : Subsystem  mask(PI DQ Stromregler){Kp=0.28*2.5/2, Ki=28*20*2, L_inv=0, Kff=0}
      mask prompts: Kp "P-Anteil:"; Ki "I-Anteil:"; L_inv "Induktivität [pu]:"; Kff "Vorsteuerung"
      mask help:
      | - in pu Einheiten
      | - 2-phasige DQ Regelung
      | - Entkopplung der d- und q-Achse
      | - Vorsteuerung der Kondensatorspannung
      | - Aktive Dämpfung der LC-Filter Resonanz
      | - Aktive Dämpfung der Zwischenkreis Spannung
  ramp2 : Constant
  u_dq0_out : Outport
  CC : Outport  Port=2
  wires:
  CC_switch/1(CC) -> CC/1, Switch/2, Logical Operator4/1, i_dq_ctrl/Enable, i_dq_ctrl/2(enable_cc), MinMax2/2
  Gain2/1 -> PhN->ab2/1
  Demux3/3 -> Terminator3/1
  Step2/1 -> Product6/1
  Data Type Conversion5/1 -> MinMax2/1
  1/f8/1 -> Saturation22/1, Saturation3/1, Saturation2/1
  Compare To Zero8/1 -> D Flip-Flop/1
  1/f4/1 -> Bias2/1
  Demux2/1 -> Sum3/1, Saturation Dynamic/2
  Sum1/1 -> Product10/1, Product7/1, Compare To Zero8/1
  Selector3/1 -> i_dq_ctrl/4(ms_i_inv_dq)
  Compare To Constant4/1 -> Data Type Conversion3/1
  Demux3/1 -> Product1/1, Product2/2
  diffPlim/1/1 -> Discrete-Time Integrator3/1
  CC_switch/2(sp_CC) -> Terminator6/1
  PQ/1 -> Selector1/1, CC_switch/4(<PQ_out>), Demux6/1
  Demux2/2 -> Mux2/2
  i_dq_ctrl/2(CCdiag) -> Terminator/1
  1/f5/1 -> Bias3/1
  Bias2/1 -> Relational Operator/2
  Product2/1 -> MinMax1/1
  Saturation1/1 -> i_dq_ctrl/3(sp_cc)
  MinMax/1 -> Saturation Dynamic/1
  0value1/1 -> i_dq_ctrl/6(u_inv_dq)
  u_dq0_in/1 -> Switch/3, Demux2/1
  Sum6/1 -> Product9/2
  Data Type Conversion4/1 -> Product7/2
  Compare To Constant/1 -> Logical Operator1/1
  Normalize8/1 -> CC_switch/3(<u_cap_ab0>)  "u_cap"
  Discrete-Time Integrator3/1 -> Relational Operator/1
  Unit Delay2/1 -> Logical Operator2/1, D Flip-Flop/2
  Data Type Conversion3/1 -> 1/f4/1
  Mux3/1 -> Saturation1/1
  i_dq_ctrl/1(sp_u_inv_dq) -> dq-dq2/1
  Logical Operator4/1 -> Discrete-Time Integrator3/2
  dq-dq2/1 -> Saturation/1
  calc_i_dq/2(i_q) -> Mux3/2
  Product11/1 -> Compare To Constant4/1
  Demux6/2 -> calc_i_dq/4(q)
  MinMax1/1 -> Saturation Dynamic/3
  Sum5/1 -> Product8/2
  Product6/1 -> CC_switch/5(dir_enable)
  calc_i_dq/1(i_d) -> Mux3/1
  ramp2/1 -> D Flip-Flop/3
  Selector4/1 -> i_dq_ctrl/5(u_ff_dq), Demux5/1
  Product9/1 -> Compare To Constant3/1
  Product10/1 -> Compare To Zero2/1
  Compare To Zero2/1 -> Data Type Conversion4/1
  1/f2/1 -> Sum6/1, Sum4/1, 1/f6/1, Product1/2
  Relational Operator/1 -> Logical Operator1/2
  PhN->ab2/1 -> Normalize8/1
  Demux5/2 -> calc_i_dq/2(uq)
  Compare To Constant3/1 -> Data Type Conversion5/1
  Data Type Conversion2/1 -> Sum5/2, 1/f1/1
  Sum3/1 -> Compare To Constant/1
  Selector2/1 -> CC_switch/6(i_out_ab)
  Mux2/1 -> Switch/1
  Saturation2/1 -> calc_i_dq/3(p)
  Data Type Conversion1/1 -> Sum5/1, 1/f2/1
  RoCoFpu/1 -> Product10/2
  Unit Delay1/1 -> Product6/2
  i_dq_3/1 -> CC_switch/2(<i_inv_dq0>), Selector3/1
  Demux2/3 -> Mux2/3
  Demux5/1 -> calc_i_dq/1(ud)
  MinMax2/1 -> Unit Delay1/1
  1/f6/1 -> Bias4/1
  Demux6/1 -> Terminator4/1
  Saturation/1 -> Demux3/1
  Product1/1 -> MinMax/2
  Saturation22/1 -> CC_switch/7(p_on)
  Logical Operator1/1 -> Logical Operator2/2
  1/f1/1 -> Sum6/2, Product2/1, 1/f5/1, Sum4/2
  Demux3/2 -> Terminator2/1
  D Flip-Flop/2 -> Data Type Conversion1/1
  Saturation Dynamic/1 -> Mux2/1, Sum3/2
  Product7/1 -> Product9/1, Product8/1
  Product8/1 -> Compare To Constant1/1
  Bias4/1 -> MinMax/1
  Sum4/1 -> Product11/2, Product6/3, 1/f8/1
  D Flip-Flop/1 -> Data Type Conversion2/1
  0value/1 -> i_dq_ctrl/1(Param)
  Saturation3/1 -> Product11/1
  Bias3/1 -> MinMax1/2
  Logical Operator2/1 -> CC_switch/8(sig_off)
  Compare To Constant1/1 -> Unit Delay2/1
  P_avoid/1 -> 1/f7/1
  u_dq/1 -> Selector4/1
  meas_i_inverter/1 -> CC_switch/1(i_inv_ab)
  i_out_dq/1 -> Selector2/1
  meas_u_cap/1 -> Gain2/1
  Switch/1 -> u_dq0_out/1
  1/f7/1 -> Sum1/2
  Selector1/1 -> Bias5/1
  Bias5/1 -> 1/f9/1
  diffPlim/4/1 -> Product12/2, Switch1/2
  Bias1/1 -> Product12/1
  Selector6/1 -> Bias1/1
  Product12/1 -> Switch1/1
  1/f3/1 -> Switch1/3
  1/f9/1 -> Sum1/1

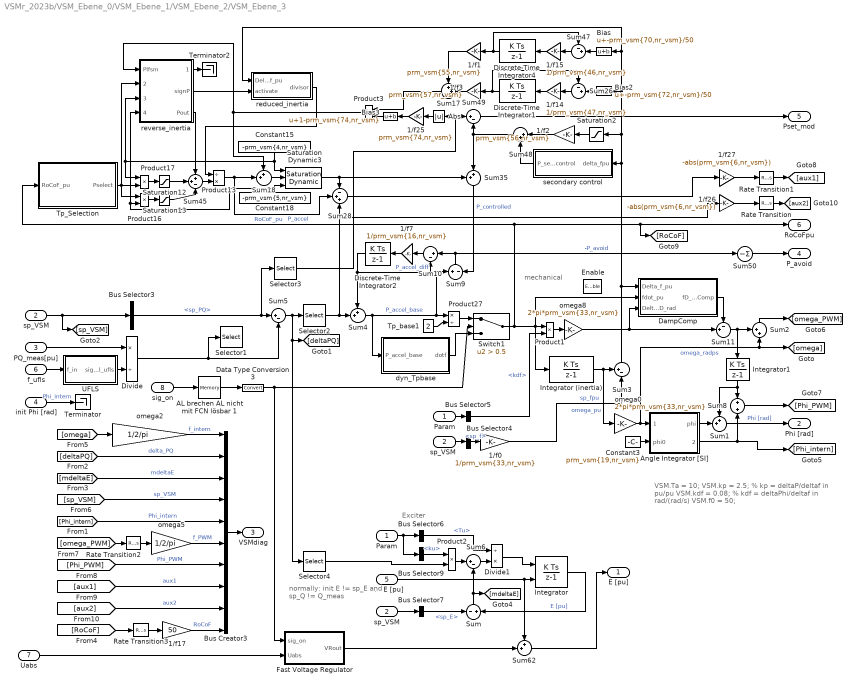
== system VSMr_2023b/VSM_Ebene_0/VSM_Ebene_1/VSM_Ebene_2/VSM_Ebene_3 ==
  note: normally:
      | init E != sp_E
      | and
      | sp_Q != Q_meas
  note: Exciter
  note: mechanical
  note: VSM.Ta = 10;
      | VSM.kp = 2.5; % kp = deltaP/deltaf  in  pu/pu
      | VSM.kdf = 0.08; % kdf = deltaPhi/deltaf in rad/(rad/s)
      | VSM.f0 = 50;
  Param : Inport
  sp_VSM : Inport  Port=2
  PQ_meas[pu] : Inport  Port=3
  init Phi [rad] : Inport  Port=4
  init E [pu] : Inport  Port=5
  f_ufls : Inport  Port=6  SampleTime=ControlSampleTime
  Uabs : Inport  Port=7  SampleTime=ControlSampleTime
  sig_on : Inport  Port=8
  Enable : EnablePort  StatesWhenEnabling=reset
  " Param " : InportShadow
  " sp_VSM " : InportShadow  Port=2
  1/f0 : Gain  Gain=1/prm_vsm{33,nr_vsm}
  1/f1 : Gain  Gain=prm_vsm{55,nr_vsm}
  1/f14 : Gain  Gain=1/prm_vsm{47,nr_vsm}
  1/f15 : Gain  Gain=1/prm_vsm{46,nr_vsm}
  1/f17 : Gain  Gain=50
  1/f2 : Gain  Gain=prm_vsm{56,nr_vsm}
  1/f25 : Gain  Gain=prm_vsm{74,nr_vsm}
  1/f26 : Gain  Gain=-abs(prm_vsm{6,nr_vsm})
  1/f27 : Gain  Gain=-abs(prm_vsm{6,nr_vsm})
  1/f3 : Gain  Gain=prm_vsm{57,nr_vsm}
  1/f7 : Gain  Gain=1/prm_vsm{16,nr_vsm}
  AL brechen AL nicht mit FCN lösbar 1 : Memory
  Abs : Abs  SaturateOnIntegerOverflow=off
  Angle Integrator [SI] : Subsystem  AncestorBlock=FriedrichLibrary/Discrete Stuff/Angle Integrator [SI]  mask{Ts=ControlSampleTime}
      mask prompts: Ts "SampleTime"
      settings: LibrarySourceBlock=FriedrichLibrary/Discrete Stuff/Angle Integrator [SI]
      mask DialogControl DescGroupVar Prompt: Angle Integrator [SI]
      mask DialogControl DescTextVar Prompt: Discrete Integrator for omega, resetting every 2*pi.
  Bias : Bias  Bias=-prm_vsm{70,nr_vsm}/50  SaturateOnIntegerOverflow=off
  Bias2 : Bias  Bias=-prm_vsm{72,nr_vsm}/50  SaturateOnIntegerOverflow=off
  Bias3 : Bias  Bias=1-prm_vsm{74,nr_vsm}  SaturateOnIntegerOverflow=off
  Bus Creator3 : BusCreator  Inputs=10
  Bus Selector3 : BusSelector  OutputSignals=sp_PQ
  Bus Selector4 : BusSelector  OutputSignals=sp_f
  Bus Selector5 : BusSelector  OutputSignals=kdf
  Bus Selector6 : BusSelector  OutputSignals=Tu
  Bus Selector7 : BusSelector  OutputSignals=sp_E
  Bus Selector9 : BusSelector  OutputSignals=ku
  Constant15 : Constant  Value=-prm_vsm{4,nr_vsm}
  Constant18 : Constant  Value=-prm_vsm{5,nr_vsm}
  Constant3 : Constant  Value=prm_vsm{19,nr_vsm}
  DampComp : Subsystem
  Data Type Conversion3 : DataTypeConversion  SaturateOnIntegerOverflow=off  RndMeth=Floor
  Discrete-Time Integrator1 : DiscreteIntegrator  gainval=1  SampleTime=-1  LimitOutput=on  UpperSaturationLimit=0  LowerSaturationLimit=prm_vsm{73,nr_vsm}/50-prm_vsm{72,nr_vsm}/50  ICPrevOutput=DiscIntNeverNeededParam  ICPrevScaledInput=DiscIntNeverNeededParam
  Discrete-Time Integrator2 : DiscreteIntegrator  gainval=1  SampleTime=-1  ICPrevOutput=DiscIntNeverNeededParam  ICPrevScaledInput=DiscIntNeverNeededParam
  Discrete-Time Integrator4 : DiscreteIntegrator  gainval=1  SampleTime=-1  LimitOutput=on  UpperSaturationLimit=prm_vsm{71,nr_vsm}/50-prm_vsm{70,nr_vsm}/50  LowerSaturationLimit=0  ICPrevOutput=DiscIntNeverNeededParam  ICPrevScaledInput=DiscIntNeverNeededParam
  Divide : Product  Inputs=*/
  Divide1 : Product  Inputs=/*
  Fast Voltage Regulator : Subsystem
  Integrator : DiscreteIntegrator  gainval=1  InitialConditionSource=external  InitialCondition=0.9  SampleTime=ControlSampleTime  ICPrevOutput=DiscIntNeverNeededParam  ICPrevScaledInput=DiscIntNeverNeededParam
  Integrator (inertia) : DiscreteIntegrator  gainval=1  InitialCondition=1  SampleTime=ControlSampleTime  LimitOutput=on  UpperSaturationLimit=prm_vsm{78,nr_vsm}  LowerSaturationLimit=prm_vsm{77,nr_vsm}  ICPrevOutput=DiscIntNeverNeededParam  ICPrevScaledInput=DiscIntNeverNeededParam
  Integrator1 : DiscreteIntegrator  gainval=1  SampleTime=ControlSampleTime  ICPrevOutput=DiscIntNeverNeededParam  ICPrevScaledInput=DiscIntNeverNeededParam
  Product{1..3,16..17} (5 alike) : Product
  Product13 : Product  Inputs=/*
  Product27 : Product  Inputs=*/
  Rate Transition{,1..3} (4 alike) : RateTransition  Integrity=off  InitialCondition=-1  OutPortSampleTime=ControlSampleTime
  Saturation Dynamic3 : simulink/Discontinuities/Saturation Dynamic  OutMin=0  OutMax=[]  OutDataTypeStr=Inherit: Same as second input  OutDataType=fixdt(1, 16)  OutScaling=2^-10  DoSatur=off
  Saturation12 : Saturate  UpperLimit=prm_vsm{38,nr_vsm}*9e9  LowerLimit=0
  Saturation13 : Saturate  UpperLimit=prm_vsm{38,nr_vsm}*9e9  LowerLimit=0
  Saturation2 : Saturate  UpperLimit=0.2/50  LowerLimit=-0.2/50
  Selector1 : Selector  InputPortWidth=2  IndexOptions=Index vector (dialog)  Indices=1  OutputSizes=1
  Selector2 : Selector  InputPortWidth=2  IndexOptions=Index vector (dialog)  Indices=1  OutputSizes=1
  Selector3 : Selector  InputPortWidth=2  IndexOptions=Index vector (dialog)  Indices=1  OutputSizes=1
  Selector4 : Selector  InputPortWidth=2  IndexOptions=Index vector (dialog)  Indices=2  OutputSizes=1
  Sum : Sum  Inputs=-|+
  Sum{1..2,4,17..18,35,62} (7 alike) : Sum  Inputs=++|
  Sum{5..6,10,49} (4 alike) : Sum  Inputs=|+-
  Sum11 : Sum  Inputs=-+|
  Sum26 : Sum  Inputs=-+|
  Sum28 : Sum  Inputs=-++
  Sum3 : Sum  Inputs=+-|
  Sum45 : Sum  Inputs=++-
  Sum47 : Sum  Inputs=-+|
  Sum48 : Sum  Inputs=|++
  Sum50 : Sum  Inputs=-
  Sum8 : Sum  Inputs=+|+
  Sum9 : Sum  Inputs=+|-
  Switch1 : Switch  Criteria=u2 > Threshold  Threshold=0.5  SaturateOnIntegerOverflow=off  InputSameDT=off
  Terminator : Terminator
  Terminator2 : Terminator
  Tp_Selection : Subsystem
  Tp_base1 : Constant  Value=2
  UFLS : Subsystem
  dyn_Tpbase : Subsystem
  omega0 : Gain  Gain=2*pi*prm_vsm{33,nr_vsm}
  omega2 : Gain  Gain=1/2/pi
  omega5 : Gain  Gain=1/2/pi
  omega8 : Gain  Gain=2*pi*prm_vsm{33,nr_vsm}
  reduced_inertia : Subsystem
  reverse_inertia : Subsystem
  secondary control : Subsystem
  "sp_VSM " : InportShadow  Port=2
  E [pu] : Outport  VectorParamsAs1DForOutWhenUnconnected=off
  Phi [rad] : Outport  Port=2  VectorParamsAs1DForOutWhenUnconnected=off
  VSMdiag : Outport  Port=3  VectorParamsAs1DForOutWhenUnconnected=off
  P_avoid : Outport  Port=4  VectorParamsAs1DForOutWhenUnconnected=off
  Pset_mod : Outport  Port=5  VectorParamsAs1DForOutWhenUnconnected=off
  RoCoFpu : Outport  Port=6  VectorParamsAs1DForOutWhenUnconnected=off
  wires:
  Sum1/1 -> Phi [rad]/1  "Phi [rad]"
  omega8/1 -> DampComp/3(Delta_fD_rad), Sum11/2
  Sum8/1 -> [Phi_PWM]
  Sum5/1 -> [deltaPQ], Selector4/1, Selector2/1
  [aux1] -> Bus Creator3/8  "aux1"
  Bus Selector4/1 -> 1/f0/1  "<sp_f>"
  Bus Selector5/1 -> Product1/2  "<kdf>"
  Bus Selector3/1 -> Sum5/1, Selector3/1  "<sp_PQ>"
  Integrator/1 -> Sum/2  "E [pu]"
  Constant3/1 -> Angle Integrator [SI]/2(phi0)
  Sum/1 -> Sum6/2, [mdeltaE]
  Angle Integrator [SI]/1(phi) -> Sum1/2
  Selector4/1 -> Product2/2
  [sp_VSM] -> Bus Creator3/4  "sp_VSM"
  Bus Selector6/1 -> Divide1/1  "<Tu>"
  Angle Integrator [SI]/2(phi_acc) -> Sum8/2, [Phi_intern]
  [deltaPQ] -> Bus Creator3/2  "delta_PQ"
  Bus Selector9/1 -> Product2/1  "<ku>"
  init Phi [rad]/1 -> Terminator/1  "Phi_intern"
  Product2/1 -> Sum6/1
  Bus Creator3/1 -> VSMdiag/1
  omega2/1 -> Bus Creator3/1  "f_intern"
  1/f0/1 -> Sum3/2  "sp_fpu"
  Sum2/1 -> [omega_PWM]
  Param/1 -> Bus Selector5/1
  [Phi_PWM] -> Bus Creator3/7  "Phi_PWM"
  [Phi_intern] -> Bus Creator3/5  "Phi_intern"
  Integrator (inertia)/1 -> Sum3/1, omega0/1  "omega_pu"
  sp_VSM/1 -> Bus Selector3/1, [sp_VSM]
  "sp_VSM "/1 -> Bus Selector4/1
  [omega] -> omega2/1
  " Param "/1 -> Bus Selector9/1, Bus Selector6/1
  [mdeltaE] -> Bus Creator3/3  "mdeltaE"
  Divide1/1 -> Integrator/1
  [aux2] -> Bus Creator3/9  "aux2"
  Bus Selector7/1 -> Sum/1  "<sp_E>"
  " sp_VSM "/1 -> Bus Selector7/1
  PQ_meas[pu]/1 -> Divide/1
  Product1/1 -> omega8/1
  Integrator1/1 -> Sum1/1, Sum8/1
  Sum6/1 -> Divide1/2
  omega0/1 -> Sum2/2, [omega], Angle Integrator [SI]/1(omega)  "omega_radps"
  DampComp/1(fD_DampComp) -> Sum11/1
  Sum4/1 -> Product27/1, Sum9/1, dyn_Tpbase/1(P_accel_base)  "P_accel_base"
  Sum10/1 -> 1/f7/1
  Discrete-Time Integrator2/1 -> Sum10/2, Sum4/1  "P_accel_diff"
  Sum3/1 -> DampComp/1(Delta_f_pu), reduced_inertia/1(Delta_f_pu), Bias/1, Bias2/1, Saturation2/1, secondary control/1(delta_fpu)
  Divide/1 -> Sum5/2, Selector1/1
  f_ufls/1 -> UFLS/1(f_in)
  UFLS/1(signal_ufls) -> Divide/2
  Switch1/1 -> Integrator (inertia)/1, DampComp/2(fdot_pu), Product1/1, RoCoFpu/1, [RoCoF], Tp_Selection/1(RoCoF_pu)  "RoCoF_pu"
  Saturation2/1 -> 1/f2/1
  Rate Transition/1 -> [aux2]
  omega5/1 -> Bus Creator3/6  "f_PWM"
  1/f7/1 -> Discrete-Time Integrator2/1
  [omega_PWM] -> Rate Transition2/1
  Rate Transition2/1 -> omega5/1
  Sum9/1 -> Sum50/1, Sum10/1  "-P_avoid"
  Selector3/1 -> Sum49/1, Abs/1
  Sum18/1 -> Saturation Dynamic3/2
  Constant15/1 -> Saturation Dynamic3/1, Product17/1, reverse_inertia/3(Plimrise)
  Product17/1 -> Saturation12/1
  Product16/1 -> Saturation13/1
  Constant18/1 -> Saturation Dynamic3/3, Product16/2, reverse_inertia/4(Plimfall)
  Saturation12/1 -> Sum45/2
  Saturation13/1 -> Sum45/3
  Product3/1 -> reverse_inertia/1(Plfsm), Sum18/1
  Sum17/1 -> Product3/1
  Sum35/1 -> Sum9/2  "P_controlled"
  Sum11/1 -> Integrator1/1, Sum2/1
  1/f14/1 -> Discrete-Time Integrator1/1
  Sum26/1 -> 1/f14/1
  Bias2/1 -> Sum26/2
  Discrete-Time Integrator1/1 -> Sum26/1, 1/f3/1
  Discrete-Time Integrator4/1 -> Sum47/1, 1/f1/1
  1/f15/1 -> Discrete-Time Integrator4/1
  Sum47/1 -> 1/f15/1
  Bias/1 -> Sum47/2
  Abs/1 -> 1/f25/1
  Sum48/1 -> Sum35/2, Sum49/2
  Sum49/1 -> Pset_mod/1
  Sum62/1 -> E [pu]/1
  init E [pu]/1 -> Integrator/2, Sum62/1
  Data Type Conversion3/1 -> Fast Voltage Regulator/1(sig_on), Switch1/2
  Tp_base1/1 -> Product27/2
  sig_on/1 -> AL brechen AL nicht mit FCN lösbar 1/1
  Rate Transition1/1 -> [aux1]
  AL brechen AL nicht mit FCN lösbar 1/1 -> Data Type Conversion3/1
  [RoCoF] -> Rate Transition3/1
  1/f17/1 -> Bus Creator3/10  "RoCoF"
  Rate Transition3/1 -> 1/f17/1
  Product27/1 -> Switch1/1
  Bias3/1 -> Product3/2
  1/f25/1 -> Bias3/1
  Sum50/1 -> P_avoid/1
  1/f1/1 -> Sum17/1
  1/f3/1 -> Sum17/2
  Sum45/1 -> Product13/2
  reverse_inertia/1(lfsm_act) -> Terminator2/1
  Product13/1 -> Sum28/2, Sum18/2  "P_accel"
  Selector2/1 -> Sum4/2, 1/f26/1, Sum28/3
  Saturation Dynamic3/1 -> Sum35/1, Sum28/1
  Sum28/1 -> 1/f27/1
  1/f27/1 -> Rate Transition1/1
  1/f26/1 -> Rate Transition/1
  Uabs/1 -> Fast Voltage Regulator/2(Uabs)
  Fast Voltage Regulator/1(VRout) -> Sum62/2
  Tp_Selection/1(Pselect) -> Product17/2, reverse_inertia/2(Pselect), Product16/1
  reverse_inertia/3(Pout) -> Sum45/1
  reverse_inertia/2(signP) -> reduced_inertia/2(activate)
  reduced_inertia/1(divisor) -> Product13/1
  dyn_Tpbase/1(dotf) -> Switch1/3
  secondary control/1(P_sec_control) -> Sum48/2
  1/f2/1 -> Sum48/1

== system VSMr_2023b/VSM_Ebene_0/VSM_Ebene_1/VSM_Ebene_2/Virtual circuit daniel style ==
  i_dq_rv : Inport
  i_dq_xv : Inport  Port=2
  Enable : EnablePort  StatesWhenEnabling=reset
  Add1 : Sum  Inputs=-+
  Add2 : Sum  Inputs=--
  Demux : Demux  Outputs=2
  Demux1 : Demux  Outputs=2
  Mux : Mux  Inputs=2
  rv : Gain  Gain=prm_vsm{14,nr_vsm}
  "rv " : Gain  Gain=prm_vsm{14,nr_vsm}
  transient rv (HP)1 : Subsystem  mask{TS=ControlSampleTime, tau=prm_vsm{13,nr_vsm}}
      mask prompts: TS "sample time"; tau "high pass time constant"
  transient rv (HP)2 : Subsystem  mask{TS=ControlSampleTime, tau=prm_vsm{13,nr_vsm}}
      mask prompts: TS "sample time"; tau "high pass time constant"
  xv : Gain  Gain=prm_vsm{15,nr_vsm}
  "xv " : Gain  Gain=prm_vsm{15,nr_vsm}
  xv1 : Gain  Gain=prm_vsm{7,nr_vsm}
  xv2 : Gain  Gain=prm_vsm{7,nr_vsm}
  v_vc_dq : Outport  VectorParamsAs1DForOutWhenUnconnected=off
  wires:
  "rv "/1 -> transient rv (HP)1/1(In1)
  transient rv (HP)2/1(Out1) -> Add2/2
  rv/1 -> transient rv (HP)2/1(In1)
  transient rv (HP)1/1(Out1) -> Add1/1
  xv2/1 -> Add2/1
  xv1/1 -> Add1/2
  "xv "/1 -> xv2/1
  xv/1 -> xv1/1
  Demux1/2 -> xv/1
  Demux1/1 -> "xv "/1
  i_dq_xv/1 -> Demux1/1
  i_dq_rv/1 -> Demux/1
  Demux/2 -> rv/1
  Add2/1 -> Mux/2
  Add1/1 -> Mux/1
  Demux/1 -> "rv "/1
  Mux/1 -> v_vc_dq/1

== system VSMr_2023b/VSM_Ebene_0/VSM_Ebene_1/VSM_Ebene_2/dq->abs ==
  In1 : Inport
  Abs : Abs  SaturateOnIntegerOverflow=off
  Demux : Demux  Outputs=3
  Real-Imag to Complex : RealImagToComplex
  Terminator : Terminator
  abs : Outport  VectorParamsAs1DForOutWhenUnconnected=off
  wires:
  Demux/3 -> Terminator/1
  Demux/1 -> Real-Imag to Complex/1
  Real-Imag to Complex/1 -> Abs/1
  In1/1 -> Demux/1
  Demux/2 -> Real-Imag to Complex/2
  Abs/1 -> abs/1

== system VSMr_2023b/VSM_Ebene_0/VSM_Ebene_1/VSM_Ebene_2/duty ==
  u_dq0 : Inport
  phi_R : Inport  Port=2
  u_dc : Inport  Port=3
  Bias : Bias  Bias=1.5*VSM.PWM.tauT*pu_vsm(nr_vsm).omegab  SaturateOnIntegerOverflow=off
  Divide : Product  Inputs=*/
  Modulation : FriedrichLibrary/Transformations/Modulation  Commented=on  Method=Sine Modulation  Ts=ControlSampleTime
  Saturation : Saturate  UpperLimit=inf  LowerLimit=1
  Subsystem : Subsystem
  dq0->ab0 phi : FriedrichLibrary/Transformations/dq0->ab0 phi  SystemSampleTime=-1  VariantActivationTime=update diagram  AllowFlexibleInterface=on  Latency=0  AutoFrameSizeCalculation=off
  d : Outport  VectorParamsAs1DForOutWhenUnconnected=off
  wires:
  phi_R/1 -> Bias/1
  u_dq0/1 -> dq0->ab0 phi/1
  Divide/1 -> Subsystem/1(AlphaBeta0)  "ab0 norm"
  dq0->ab0 phi/1 -> Divide/1
  Subsystem/1(Duty) -> d/1
  Bias/1 -> dq0->ab0 phi/2
  u_dc/1 -> Saturation/1
  Saturation/1 -> Divide/2

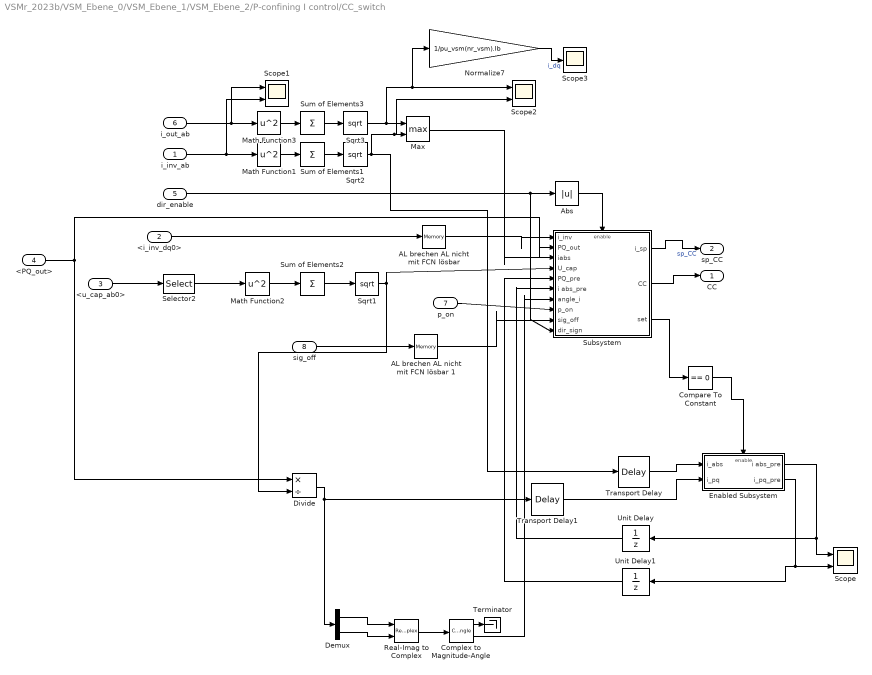
== system VSMr_2023b/VSM_Ebene_0/VSM_Ebene_1/VSM_Ebene_2/P-confining I control/CC_switch ==
  i_inv_ab : Inport
  <i_inv_dq0> : Inport  Port=2
  <u_cap_ab0> : Inport  Port=3
  <PQ_out> : Inport  Port=4
  dir_enable : Inport  Port=5
  i_out_ab : Inport  Port=6
  p_on : Inport  Port=7
  sig_off : Inport  Port=8
  "AL brechen AL nicht mit FCN lösbar " : Memory
  AL brechen AL nicht mit FCN lösbar 1 : Memory
  Abs : Abs  SaturateOnIntegerOverflow=off
  Compare To Constant : simulink/Logic and Bit Operations/Compare To Constant  relop===  const=0  OutDataTypeStr=boolean
  Complex to Magnitude-Angle : ComplexToMagnitudeAngle
  Demux : Demux  Outputs=2
  Divide : Product  Inputs=*/
  Enabled Subsystem : Subsystem  TreatAsAtomicUnit=on
  Math Function1 : Math  Operator=square  SignedPower=on
  Math Function2 : Math  Operator=square  SignedPower=on
  Math Function3 : Math  Operator=square  SignedPower=on
  Max : MinMax  Function=max  Inputs=2
  Normalize7 : Gain  Gain=1/pu_vsm(nr_vsm).Ib  OutDataTypeStr=double  RndMeth=Round
  Real-Imag to Complex : RealImagToComplex
  Scope : Scope  NumInputPorts=2
  Scope1 : Scope  NumInputPorts=2
  Scope2 : Scope  NumInputPorts=2
  Scope3 : Scope
  Selector2 : Selector  InputPortWidth=3  IndexOptions=Index vector (dialog)  Indices=[1 2]  OutputSizes=1
  Sqrt1 : Sqrt
  Sqrt2 : Sqrt
  Sqrt3 : Sqrt
  Subsystem : Subsystem
  Sum of Elements1 : Sum  Inputs=+
  Sum of Elements2 : Sum  Inputs=+
  Sum of Elements3 : Sum  Inputs=+
  Terminator : Terminator
  Transport Delay : TransportDelay  DelayTime=0.1
  Transport Delay1 : TransportDelay  DelayTime=0.1
  Unit Delay : UnitDelay  SampleTime=ControlSampleTime  HasFrameUpgradeWarning=on
  Unit Delay1 : UnitDelay  SampleTime=ControlSampleTime  HasFrameUpgradeWarning=on
  CC : Outport
  sp_CC : Outport  Port=2
  wires:
  Sum of Elements1/1 -> Sqrt2/1
  Selector2/1 -> Math Function2/1
  Math Function1/1 -> Sum of Elements1/1
  Sum of Elements2/1 -> Sqrt1/1
  "AL brechen AL nicht mit FCN lösbar "/1 -> Subsystem/1(i_inv)
  Sqrt1/1 -> Subsystem/4(U_cap), Divide/2
  Math Function2/1 -> Sum of Elements2/1
  <u_cap_ab0>/1 -> Selector2/1
  <i_inv_dq0>/1 -> "AL brechen AL nicht mit FCN lösbar "/1
  Subsystem/1(i_sp) -> sp_CC/1  "sp_CC"
  i_inv_ab/1 -> Scope1/2, Math Function1/1
  Subsystem/2(CC) -> CC/1
  <PQ_out>/1 -> Divide/1, Subsystem/2(PQ_out)
  dir_enable/1 -> Subsystem/10(dir_sign), Abs/1
  Compare To Constant/1 -> Enabled Subsystem/Enable
  Enabled Subsystem/1(i abs_pre) -> Scope/1, Unit Delay/1
  Subsystem/3(set) -> Compare To Constant/1
  Transport Delay/1 -> Enabled Subsystem/1(i_abs)
  Unit Delay/1 -> Subsystem/6(i abs_pre)
  Enabled Subsystem/2(i_pq_pre) -> Unit Delay1/1, Scope/2
  Unit Delay1/1 -> Subsystem/5(PQ_pre)
  Transport Delay1/1 -> Enabled Subsystem/2(i_pq)
  Math Function3/1 -> Sum of Elements3/1
  Sum of Elements3/1 -> Sqrt3/1
  i_out_ab/1 -> Scope1/1, Math Function3/1
  Sqrt3/1 -> Normalize7/1, Scope2/1, Max/1
  Sqrt2/1 -> Scope2/2, Max/2, Transport Delay/1
  Max/1 -> Subsystem/3(iabs)
  Demux/1 -> Real-Imag to Complex/1
  Demux/2 -> Real-Imag to Complex/2
  Divide/1 -> Demux/1, Transport Delay1/1
  Real-Imag to Complex/1 -> Complex to Magnitude-Angle/1
  Complex to Magnitude-Angle/2 -> Subsystem/7(angle_i)
  Normalize7/1 -> Scope3/1  "i_dq"
  p_on/1 -> Subsystem/8(p_on)
  sig_off/1 -> AL brechen AL nicht mit FCN lösbar 1/1
  AL brechen AL nicht mit FCN lösbar 1/1 -> Subsystem/9(sig_off)
  Abs/1 -> Subsystem/Enable
  Complex to Magnitude-Angle/1 -> Terminator/1
